simulink model "lab5"  (R2020b)
settings: Solver=VariableStepAuto  StartTime=0.0  StopTime=10.0  RelTol=1e-3
libraries: dspsnks4 x1, dspvision x1, dspsigops x1
settings Model: Creator=superdeano  LastModifiedBy=superdeano

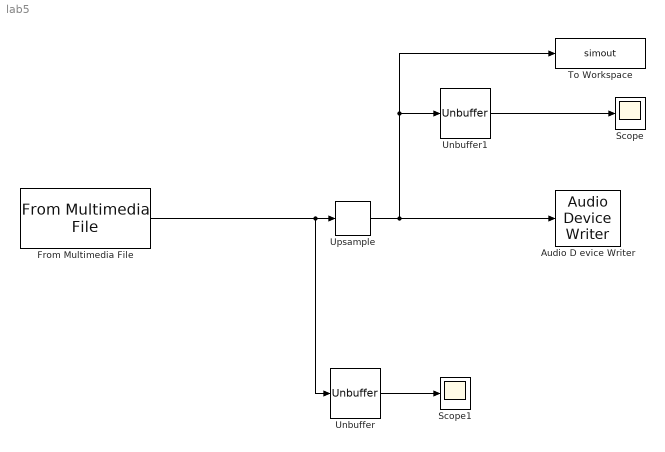
== system lab5 ==
  Audio D evice Writer : dspsnks4/Audio Device Writer  Driver=CoreAudio  Device=Default  InheritSampleRate=on  SampleRate=44100  BitDepth=16-bit integer  BufferSize=4096  NumBuffers=10  DefaultOutputChannelMapping=on  OutputChannelMapping=1:2  OutputNumUnderrunSamples=off  DriverIdx=5  DeviceWarnFlag=''
  From Multimedia File : dspvision/From Multimedia File  inputFilename=/Users/superdeano/Documents/GitHub/MATLAB/ELEC 342/Lab 5/ELEC_364_lab_5_Audio_S.wav  readRange=[1 Inf]  loop=on  numPlays=inf  outputStreams=Audio only  videoDataType=single  audioDataType=double  inheritSampleTime=on  userDefinedSampleTime=1/30  noAudioOutput=off  isIntensityVideo=off  fourcc=RGB  colorVideoFormat=Separate color signals  outputEOF=off  dataOrg=Column-major  audioFrameSize=1024  computeAudioFrameSize=off  outSamplingMode=Sample based
  Scope : Scope
  Scope1 : Scope
  To Workspace : ToWorkspace  VariableName=simout  SaveFormat=Timeseries  SampleTime=-1
      settings: MaxDataPoints=327680
  Unbuffer : Unbuffer
  Unbuffer1 : Unbuffer
  Upsample : dspsigops/Upsample  N=1  phase=0  InputProcessing=Columns as channels (frame based)  RateOptions=Enforce single-rate processing  ic=0  mode=Unused parameter value
  wires:
  From Multimedia File/1 -> Upsample/1, Unbuffer/1
  Unbuffer/1 -> Scope1/1
  Upsample/1 -> To Workspace/1, Unbuffer1/1, Audio D evice Writer/1
  Unbuffer1/1 -> Scope/1
